simulink model "single_phase_matrix_converter"  (R2016b)
settings: Solver=VariableStepAuto  StartTime=0.0  StopTime=1  RelTol=1e-3
libraries: powerlib x15
settings Model: Creator=CNK  LastModifiedBy=CNK

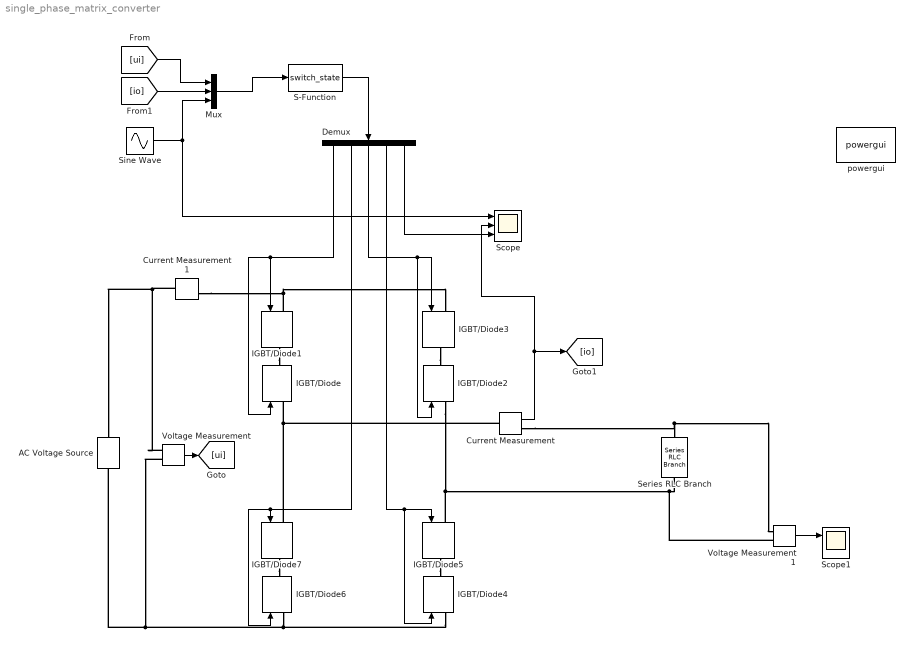
== system single_phase_matrix_converter ==
  AC Voltage Source : powerlib/Electrical Sources/AC Voltage Source  Amplitude=100  Phase=0  Frequency=50  SampleTime=0  Measurements=None  BusType=swing  Pref=10e3  Qref=0  Qmin=-inf  Qmax=+inf
  Current Measurement : powerlib/Measurements/Current Measurement  PhasorSimulation=off  OutputType=Complex  PSBequivalent=0
  Current Measurement1 : powerlib/Measurements/Current Measurement  PhasorSimulation=off  OutputType=Complex  PSBequivalent=0
  Demux : Demux  Outputs=5
  IGBT/Diode{,1..7} (8 alike) : powerlib/Power Electronics/IGBT//Diode  Ron=1e-3  Rs=1e5  Cs=inf  Measurements=off
  Mux : Mux  Inputs=3
  S-Function : S-Function  FunctionName=switch_state  SFunctionDeploymentMode=off  EnableBusSupport=off
  Scope : Scope  NumInputPorts=3
  Scope1 : Scope  NumInputPorts=2
  Series RLC Branch : powerlib/Elements/Series RLC Branch  LConnTagsString=__new0  RConnTagsString=__new0  BranchType=RL  Resistance=2  Inductance=0.04  SetiL0=off  InitialCurrent=0  Capacitance=1e-6  Setx0=off  InitialVoltage=0  Measurements=None
  Sine Wave : Sin  Amplitude=5  Frequency=100  SampleTime=0
  Voltage Measurement : powerlib/Measurements/Voltage Measurement  PhasorSimulation=off  OutputType=Complex  PSBequivalent=0
  Voltage Measurement1 : powerlib/Measurements/Voltage Measurement  PhasorSimulation=off  OutputType=Complex  PSBequivalent=0
  powergui : powerlib/powergui  Priority=1  SimulationMode=Continuous  SolverType=Tustin/Backward Euler (TBE)  SampleTime=50e-6  frequency=60  SPID=off  DisableSnubberDevices=off  DisableRonSwitches=off  DisableVfSwitches=off  SwTol=0  DisplayEquations=off  Interpol=off  ExternalGateDelay=off  methode=off  Ts=10  FunctionMessages=off  echomessages=off  HookPort=off  EnableUseOfTLC=off  x0status=blocks  frequencyindice=50  Pbase=100e6  ErrMax=1e-4  Iterations=50  UnitsV=kV  UnitsW=MW  buscounter=0  RestoreLinks=warning  ResistiveCurrentMeasurement=off  Frange=[0:2:500]  Ylog=off  Xlog=on  ShowGrid=off  save=off  variable=ZData  structure=0  ZoomFFT=off  StartTime=0.0  cycles=1  DisplayStyle=1  fundamental=60  FreqAxis=off  MaxFrequency=1000  frequencyindicesteady=1  RmsSteady=1  display=off
  wires:
  Demux/1 -> IGBT/Diode/1, IGBT/Diode1/1
  Demux/2 -> IGBT/Diode6/1, IGBT/Diode7/1
  Demux/4 -> IGBT/Diode4/1, IGBT/Diode5/1
  Demux/3 -> IGBT/Diode2/1, IGBT/Diode3/1
  Current Measurement/1 -> [io], Scope/2
  Voltage Measurement1/1 -> Scope1/1
  Voltage Measurement/1 -> [ui]
  [io] -> Mux/2
  [ui] -> Mux/1
  Mux/1 -> S-Function/1
  S-Function/1 -> Demux/1
  Sine Wave/1 -> Scope/1, Mux/3
  Demux/5 -> Scope/3
  connections:
  IGBT/Diode1/RConn1 -- IGBT/Diode/RConn1
  IGBT/Diode3/RConn1 -- IGBT/Diode2/RConn1
  IGBT/Diode5/RConn1 -- IGBT/Diode4/RConn1
  IGBT/Diode7/RConn1 -- IGBT/Diode6/RConn1
  IGBT/Diode2/LConn1 -- IGBT/Diode5/LConn1 -- Series RLC Branch/RConn1 -- Voltage Measurement1/LConn2
  IGBT/Diode7/LConn1 -- Current Measurement/LConn1 -- IGBT/Diode/LConn1
  Voltage Measurement/LConn1 -- Current Measurement1/LConn1 -- AC Voltage Source/RConn1
  IGBT/Diode6/LConn1 -- AC Voltage Source/LConn1 -- Voltage Measurement/LConn2 -- IGBT/Diode4/LConn1
  Current Measurement/RConn1 -- Voltage Measurement1/LConn1 -- Series RLC Branch/LConn1
  IGBT/Diode1/LConn1 -- Current Measurement1/RConn1 -- IGBT/Diode3/LConn1
